simulink model "Fuzzy_pitch_angle"  (R2014a)
settings: Solver=ode23  StartTime=0.0  StopTime=40  RelTol=1e-3
undefined symbols (not defined in the file): C01, C1, Cd, Ce, fuzzy_PI
libraries: fuzblock x1
settings Model: Creator=nnn  LastModifiedBy=nnn
settings SolverCC: ZeroCrossControl=DisableAll  AutoInsertRateTranBlk=on

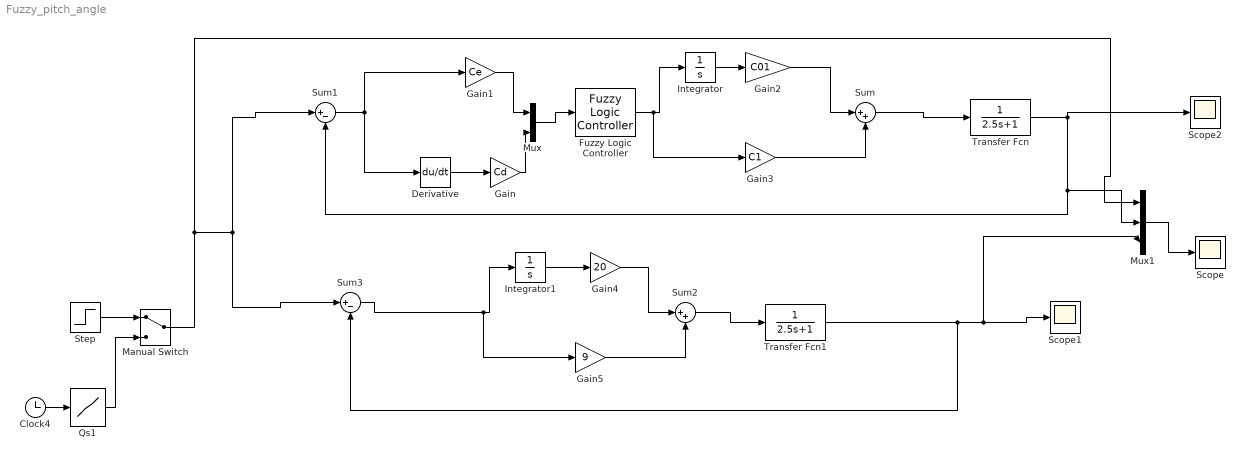
== system Fuzzy_pitch_angle ==
  Clock4 : Clock
      settings: Decimation=100
  Derivative : Derivative
  Fuzzy Logic Controller : fuzblock/Fuzzy Logic  Controller  fis=[fuzzy_PI]
  Gain : Gain  Gain=Cd
  Gain1 : Gain  Gain=Ce
  Gain2 : Gain  Gain=C01
  Gain3 : Gain  Gain=C1
  Gain4 : Gain  Gain=20
  Gain5 : Gain  Gain=9
  Integrator : Integrator
  Integrator1 : Integrator
  Manual Switch : ManualSwitch
  Mux : Mux  Inputs=2
  Mux1 : Mux  Inputs=3
  Qs1 : Lookup  InputValues=[0 20 25 30]  Table="[0 0  1.0 1.0]"  SaturateOnIntegerOverflow=on
  Scope : Scope
  Scope1 : Scope
  Scope2 : Scope
      settings: YMin=0.75  YMax=1.5  SaveName=ScopeData2
  Step : Step  SampleTime=0
  Sum : Sum  Inputs=|++
  Sum1 : Sum  Inputs=|+-
  Sum2 : Sum  Inputs=|++
  Sum3 : Sum  Inputs=|+-
  Transfer Fcn : TransferFcn  Denominator=[2.5 1]
  Transfer Fcn1 : TransferFcn  Denominator=[2.5 1]
  wires:
  Derivative/1 -> Gain/1
  Gain/1 -> Mux/2
  Mux/1 -> Fuzzy Logic Controller/1
  Sum1/1 -> Gain1/1, Derivative/1
  Gain1/1 -> Mux/1
  Integrator/1 -> Gain2/1
  Fuzzy Logic Controller/1 -> Gain3/1, Integrator/1
  Sum2/1 -> Transfer Fcn1/1
  Integrator1/1 -> Gain4/1
  Gain4/1 -> Sum2/1
  Sum3/1 -> Gain5/1, Integrator1/1
  Gain5/1 -> Sum2/2
  Mux1/1 -> Scope/1
  Transfer Fcn/1 -> Mux1/2, Sum1/2, Scope2/1
  Gain3/1 -> Sum/2
  Gain2/1 -> Sum/1
  Manual Switch/1 -> Mux1/1, Sum1/1, Sum3/1
  Transfer Fcn1/1 -> Mux1/3, Scope1/1, Sum3/2
  Clock4/1 -> Qs1/1
  Step/1 -> Manual Switch/1
  Qs1/1 -> Manual Switch/2
  Sum/1 -> Transfer Fcn/1
